simulink model "env_extQ16"  (R2022b)
settings: Solver=VariableStepAuto  StartTime=0.0  StopTime=30  RelTol=1e-3
values from neighbouring files (symbols this model uses):
  B = 8    [variables.m]    (also in variables16.m)
  cordic_delay = 20    [variables.m]    (also in variables16.m)
  e_val = 1/l2    [variables.m]    (also in variables16.m)
  exp_fract_len_homo = 26    [variables.m]    (also in variables16.m = 10)
  exp_word_len_homo = 32    [variables.m]    (also in variables16.m = 16)
  explarge_delay = 3    [variables.m]    (also in variables16.m)
  fft_len_hilb = 2048    [variables.m]    (also in variables16.m)
  fft_length = 4096    [variables.m]    (also in variables16.m)
  frac_bit_l2 = 30    [variables.m]    (also in variables16.m = 14)
  frac_bit_l3 = 29    [variables.m]    (also in variables16.m = 13)
  frac_bit_l4 = 28    [variables.m]    (also in variables16.m = 12)
  grp_delay_hilb = 11    [variables.m]    (also in variables16.m)
  grp_delay_homo = 13    [variables.m]    (also in variables16.m)
  grp_delay_psd = 19    [variables.m]    (also in variables16.m)
  grp_delay_swt = 12    [variables.m]    (also in variables16.m)
  l2 = log(2)    [variables.m]    (also in variables16.m)
  l2e = 1/log2(exp(1))    [variables.m]    (also in variables16.m)
  log2_table = log2((2^(B-1) : 2^(B)) / 2^(B - 1))    [variables.m]    (also in variables16.m)
  log_fract_len_homo = 31    [variables.m]    (also in variables16.m = 15)
  log_latency = 21    [variables.m]    (also in variables16.m)
  log_word_len = 48    [variables.m]    (also in variables16.m = 24)
  log_word_len_homo = 32    [variables.m]    (also in variables16.m = 16)
  NLZLUT = B-ceil(log2((1:2^B)))    [variables.m]    (also in variables16.m)
  scale = 1.0 / (fs * sum(window_val.*window_val))    [variables.m]    (also in variables16.m)
  win_dim = 64    [variables.m]    (also in variables16.m)
  window_dim = 100    [variables.m]    (also in variables16.m)
undefined symbols (not defined in the file or in its folder): C, c, fl_high_index, fl_low_index, HiD, hilbert_fifo_full, LoD, psd_fifo_full, SFVC784, swt_fifo_full, XCK26, xlfda_numerator
libraries: hdlBasic x626, hdlDSPIP x12, hdlUtilities x2, dspsnks4 x1, dspvision x1, vmcUtilities x1
(part 1 of 7)
settings Model: Creator=windows  LastModifiedBy=domen
settings DataIOCC: SaveTime=off

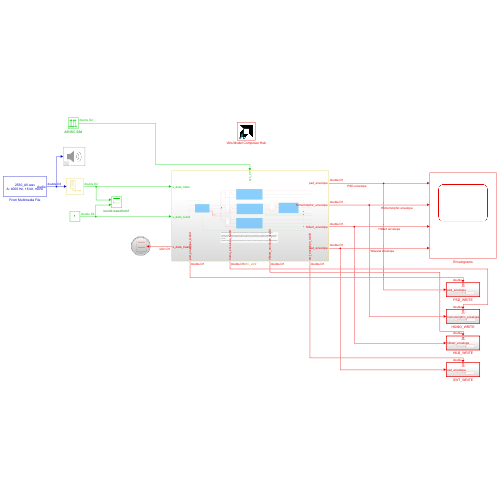
[thumbnail: Simulink's stored preview of the top-level diagram]
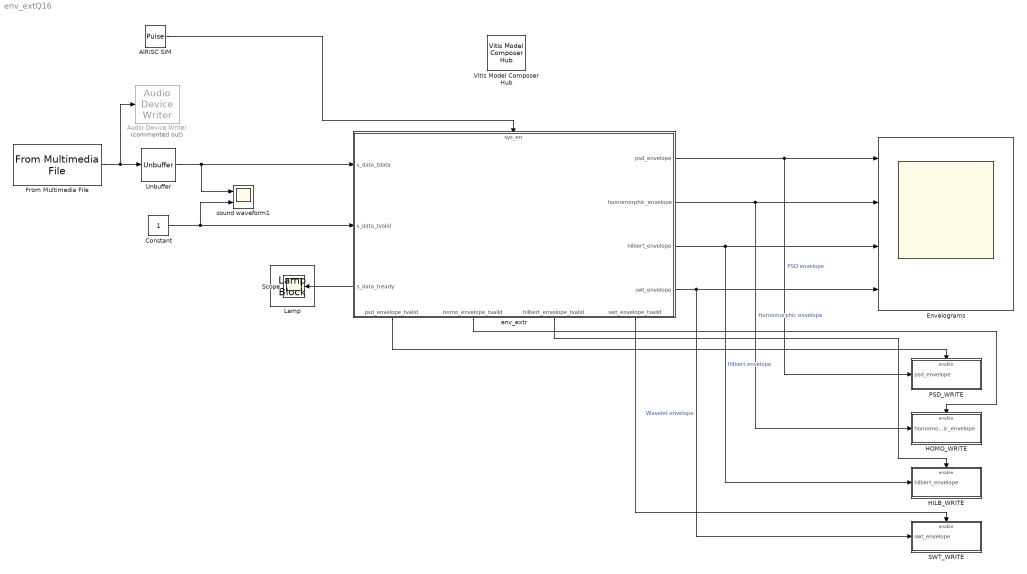
== system env_extQ16 ==
  AIRISC SIM : DiscretePulseGenerator  Period=5120  PulseWidth=2560  PhaseDelay=6144  SampleTime=1/4e3
  Audio Device Writer : dspsnks4/Audio Device Writer  Commented=on  Driver=DirectSound  Device=Default  InheritSampleRate=on  SampleRate=44100  BitDepth=16-bit integer  BufferSize=4096  NumBuffers=10  DefaultOutputChannelMapping=on  OutputChannelMapping=1:2  OutputNumUnderrunSamples=off  DriverIdx=1  DeviceWarnFlag=''
  Constant : Constant  SampleTime=1/4e3
  Envelograms : Scope  NumInputPorts=4
  From Multimedia File : dspvision/From Multimedia File  inputFilename=C:\hss_tests\2530_AV.wav  readRange=[1 Inf]  loop=on  numPlays=1  outputStreams=Audio only  videoDataType=single  audioDataType=double  inheritSampleTime=on  userDefinedSampleTime=1/4  noAudioOutput=off  isIntensityVideo=off  fourcc=RGB  colorVideoFormat=Separate color signals  outputEOF=off  dataOrg=Column-major  audioFrameSize=1024  computeAudioFrameSize=off  outSamplingMode=Sample based
      settings: LibrarySourceBlock=dspsrcs4/From Multimedia File
  HILB_WRITE : Subsystem  TreatAsAtomicUnit=on
  HOMO_WRITE : Subsystem  TreatAsAtomicUnit=on
  Lamp : LampBlock  LabelPosition=Hide
  PSD_WRITE : Subsystem  TreatAsAtomicUnit=on
  SWT_WRITE : Subsystem  TreatAsAtomicUnit=on
  Scope : Scope
  Unbuffer : Unbuffer
  Vitis Model Composer Hub : vmcUtilities/Vitis Model Composer Hub  Tag=genX  CodeGeneration=off  SubsystemName=env_extr  TargetDirectory=./code  ExportType=AI Engines  IpVendor=xilinx.com  IpLibrary=hls  IpVersion=1.0  IpHWLanguage=Verilog  AieCompilerOptions={}  AieSimulatorOptions={}  CreateTestbench=off  TestbenchStackSize=10  RunRtlSim=off  RunCSim=off  RunAieSim=off  AieSimTimeout=50000  RunAieSimProfiling=off  LaunchVitisAnalyzer=off  PlotOutput=off  RunX86Sim=off  X86SimTimeout=10  GenHwImage=off  GenLibadfXo=off  PlatformType=Not Specified  HwSystemType=Baremetal  HwValidationTarget=hw  ProjDevice=Kria KV260 Vision AI Starter Kit (xck26-sfvc784-2LV-c)  ProjDevicePart=XCK26-SFVC784-2LV-C  AIEType=None  SamplePeriod=-1  ClockFrequency=200  DataPathParallelism=1  xilinxfamily=zynquplus  part=xck26  speed=-2LV-c  package=sfvc784  directory=./code\ip\env_extr\src  testbench=off  incr_netlist=off  synthesis_tool=Vivado  clock_wrapper=Clock Enables  dbl_ovrd=According to Block Masks  dcm_input_clock_period=10  sysclk_period=1e9/1e6  simulink_period=1/1e6  eval_field=0  LogFileName=''  NThreads=4
  env_extr : Subsystem
      settings: PortSchema="{\"entries\":[{\"content\":{\"sides\":[{\"content\":{\"connectorIds\":[\"In1\",\"In2\",\"Out9\"]},\"type\":\"ConnectorPlacement.EquallySpacedRectSide\",\"uuid\":\"43992d7e-e6ac-477d-8ccd-89dbeb08d59b\"},{\"content\":{\"connectorIds\":[\"Out1\",\"Out2\",\"Out3\",\"Out4\"],\"side\":\"RIGHT\"},\"type\":\"ConnectorPlacement.EquallySpacedRectSide\",\"uuid\":\"9fd35b87-a22a-4e27-bfaa-04533d92a615\"},{\"content\":{\"connectorIds\":[\"In3\"],\"side\":\"TOP\"},\"type\":\"ConnectorPlacement.EquallySpacedRectSide\",\"uuid\":\"ce144599-82ea-4426-8dad-840a4d497276\"},{\"content\":{\"connectorIds\":[\"Out5\",\"Out6\",\"Out7\",\"Out8\"],\"side\":\"BOTTOM\"},\"type\":\"ConnectorPlacement.EquallySpacedRectSide\",\"uuid\":\"d757f4f1-9e3b-423a-82f0-618de1a239f4\"}]},\"type\":\"ConnectorPlacement.EquallySpacedConnector\",\"uuid\":\"098bbe0e-14d9-4fd5-a746-b1683e211a6b\"}],\"packageUris\":[\"http://schema.mathworks.com/mf0/Connector/R2020b\"],\"version\":\"1.0\"}"
  sound waveform1 : Scope  NumInputPorts=2
  wires:
  env_extr/2(homomorphic_envelope) -> HOMO_WRITE/1(homomorphic_envelope), Envelograms/2  "Homomorphic envelope"
  From Multimedia File/1 -> Unbuffer/1, Audio Device Writer/1
  Unbuffer/1 -> sound waveform1/1, env_extr/1(s_data_tdata)
  env_extr/4(swt_envelope) -> SWT_WRITE/1(swt_envelope), Envelograms/4  "Wavelet envelope"
  env_extr/1(psd_envelope) -> PSD_WRITE/1(psd_envelope), Envelograms/1  "PSD envelope"
  env_extr/3(hilbert_envelope) -> HILB_WRITE/1(hilbert_envelope), Envelograms/3  "Hilbert envelope"
  Constant/1 -> sound waveform1/2, env_extr/2(s_data_tvalid)
  env_extr/9(s_data_tready) -> Scope/1
  env_extr/8(swt_envelope_tvalid) -> SWT_WRITE/Enable
  env_extr/7(hilbert_envelope_tvalid) -> HILB_WRITE/Enable
  env_extr/6(homo_envelope_tvalid) -> HOMO_WRITE/Enable
  env_extr/5(psd_envelope_tvalid) -> PSD_WRITE/Enable
  AIRISC SIM/1 -> env_extr/3(sys_en)

== system env_extQ16/HILB_WRITE ==
  hilbert_envelope : Inport
  Enable : EnablePort
  To Workspace : ToWorkspace  VariableName=hilb_envelope  SampleTime=-1
  wires:
  hilbert_envelope/1 -> To Workspace/1

== system env_extQ16/HOMO_WRITE ==
  homomorphic_envelope : Inport
  Enable : EnablePort
  To Workspace1 : ToWorkspace  VariableName=homo_envelope  SampleTime=-1
  wires:
  homomorphic_envelope/1 -> To Workspace1/1

== system env_extQ16/PSD_WRITE ==
  psd_envelope : Inport
  Enable : EnablePort
  To Workspace3 : ToWorkspace  VariableName=psd_envelope  SampleTime=-1
  wires:
  psd_envelope/1 -> To Workspace3/1

== system env_extQ16/SWT_WRITE ==
  swt_envelope : Inport
  Enable : EnablePort
  To Workspace2 : ToWorkspace  VariableName=swt_envelope  SampleTime=-1
  wires:
  swt_envelope/1 -> To Workspace2/1

== system env_extQ16/env_extr ==
  note: This "feature extractor" system can used to perform the pre-procesing of incoming PCG audio signal.
      |
      | In particular, after a noise removal pre-filtering, it performs, in parallel and in a pipeline fashion, the extraction of four features, namely the PSD envelope, the Hilbert envelope, the Homomorphic envelope and the SWT envelope.
      |
      | The details about the operations performed can be found here: https://ieeexplore.ieee.org/document/7234876
  s_data_tdata : Inport
  s_data_tvalid : Inport  Port=2
  sys_en : Inport  Port=3
  Bus Creator : BusCreator  Inputs=psd_fifo_full,hilbert_fifo_full,swt_fifo_full
  FIFO : hdlBasic/FIFO  mem_type=Block RAM  performance_options=Standard_FIFO  embedded_registers=off  depth=8K  use_asym_data_widths=off  asym_read_width=32  percent_nbits=1  rst=off  rst_latency=2  en=off  use_dcount=off  use_percent_full_port=off  use_almost_empty=off  almost_empty_thresh=3  use_almost_full=off  use_rd_rst_busy=off  use_wr_rst_busy=off  almost_full_thresh=14  almost_empty_offset=[]  almost_full_offset=[]  explicit_period=off  period=[]  store_only_valid=[]  init_zero=[]  simulation_type=fast_sim  XmcBlockStatus=1  maskContainerNames=tabcontainer1  block_type=fifo  block_config=sysgen:FIFO_config  block_width=538  block_height=997
      settings: infoedit=[]
  FIFO1 : hdlBasic/FIFO  mem_type=Block RAM  performance_options=Standard_FIFO  embedded_registers=off  depth=8K  use_asym_data_widths=off  asym_read_width=32  percent_nbits=1  rst=off  rst_latency=2  en=off  use_dcount=off  use_percent_full_port=off  use_almost_empty=off  almost_empty_thresh=2  use_almost_full=off  use_rd_rst_busy=off  use_wr_rst_busy=off  almost_full_thresh=14  almost_empty_offset=[]  almost_full_offset=[]  explicit_period=off  period=[]  store_only_valid=[]  init_zero=[]  simulation_type=fast_sim  XmcBlockStatus=1  maskContainerNames=tabcontainer1  block_type=fifo  block_config=sysgen:FIFO_config  block_width=538  block_height=997
      settings: infoedit=[]
  FIFO2 : hdlBasic/FIFO  mem_type=Block RAM  performance_options=Standard_FIFO  embedded_registers=off  depth=8K  use_asym_data_widths=off  asym_read_width=32  percent_nbits=1  rst=off  rst_latency=2  en=off  use_dcount=off  use_percent_full_port=off  use_almost_empty=off  almost_empty_thresh=3  use_almost_full=off  use_rd_rst_busy=off  use_wr_rst_busy=off  almost_full_thresh=14  almost_empty_offset=[]  almost_full_offset=[]  explicit_period=off  period=[]  store_only_valid=[]  init_zero=[]  simulation_type=fast_sim  XmcBlockStatus=1  maskContainerNames=tabcontainer1  block_type=fifo  block_config=sysgen:FIFO_config  block_width=538  block_height=997
      settings: infoedit=[]
  FIFO3 : hdlBasic/FIFO  mem_type=Block RAM  performance_options=Standard_FIFO  embedded_registers=off  depth=8K  use_asym_data_widths=off  asym_read_width=32  percent_nbits=1  rst=off  rst_latency=2  en=off  use_dcount=off  use_percent_full_port=off  use_almost_empty=off  almost_empty_thresh=1  use_almost_full=off  use_rd_rst_busy=off  use_wr_rst_busy=off  almost_full_thresh=8190  almost_empty_offset=[]  almost_full_offset=[]  explicit_period=off  period=[]  store_only_valid=[]  init_zero=[]  simulation_type=fast_sim  XmcBlockStatus=1  maskContainerNames=tabcontainer1  block_type=fifo  block_config=sysgen:FIFO_config  block_width=538  block_height=997
      settings: infoedit=[]
  FILTERING : Subsystem
      settings: PortSchema="{\"entries\":[{\"content\":{\"sides\":[{\"content\":{\"connectorIds\":[\"In1\",\"In2\",\"Out4\"]},\"type\":\"ConnectorPlacement.EquallySpacedRectSide\",\"uuid\":\"9d039a16-3a48-49d5-80b7-ade04a8e7f96\"},{\"content\":{\"connectorIds\":[\"Out1\",\"Out2\",\"In4\"],\"side\":\"RIGHT\"},\"type\":\"ConnectorPlacement.EquallySpacedRectSide\",\"uuid\":\"bb4be220-296c-4d2d-b90e-a958a467eb47\"},{\"content\":{\"connectorIds\":[\"In3\"],\"side\":\"TOP\"},\"type\":\"ConnectorPlacement.EquallySpacedRectSide\",\"uuid\":\"bb4a24ca-25c4-4b34-8f6b-74df8c85655a\"},{\"content\":{\"connectorIds\":[\"Out3\"],\"side\":\"BOTTOM\"},\"type\":\"ConnectorPlacement.EquallySpacedRectSide\",\"uuid\":\"f96279e1-557f-4274-b1c8-f07939b904f6\"}]},\"type\":\"ConnectorPlacement.EquallySpacedConnector\",\"uuid\":\"a2ca7259-7cd6-4f5b-b082-7ba40fce56a8\"}],\"packageUris\":[\"http://schema.mathworks.com/mf0/Connector/R2020b\"],\"version\":\"1.0\"}"
  HILBERT : Subsystem
      settings: PortSchema="{\"entries\":[{\"content\":{\"sides\":[{\"content\":{\"connectorIds\":[\"In1\",\"In2\",\"Out5\"]},\"type\":\"ConnectorPlacement.EquallySpacedRectSide\",\"uuid\":\"c096cd28-364f-4c7f-b687-c45e0f672067\"},{\"content\":{\"connectorIds\":[\"Out1\",\"Out2\",\"In3\",\"Out3\",\"Out4\",\"In4\"],\"side\":\"RIGHT\"},\"type\":\"ConnectorPlacement.EquallySpacedRectSide\",\"uuid\":\"8f6de1f0-0c6d-47b5-8720-be9e335b7472\"},{\"content\":{\"connectorIds\":[],\"side\":\"TOP\"},\"type\":\"ConnectorPlacement.EquallySpacedRectSide\",\"uuid\":\"cb0bdd80-75cb-433b-a701-3f68d903d9bd\"}]},\"type\":\"ConnectorPlacement.EquallySpacedConnector\",\"uuid\":\"0550c3cb-50ae-4da2-a768-6cf438586d1d\"}],\"packageUris\":[\"http://schema.mathworks.com/mf0/Connector/R2020b\"],\"version\":\"1.0\"}"
  HOMOMORPHIC : Subsystem
      settings: PortSchema="{\"entries\":[{\"content\":{\"sides\":[{\"content\":{\"connectorIds\":[\"In1\",\"In2\",\"Out3\"]},\"type\":\"ConnectorPlacement.EquallySpacedRectSide\",\"uuid\":\"9d039a16-3a48-49d5-80b7-ade04a8e7f96\"},{\"content\":{\"connectorIds\":[\"Out1\",\"Out2\",\"In3\"],\"side\":\"RIGHT\"},\"type\":\"ConnectorPlacement.EquallySpacedRectSide\",\"uuid\":\"bb4be220-296c-4d2d-b90e-a958a467eb47\"},{\"content\":{\"connectorIds\":[],\"side\":\"TOP\"},\"type\":\"ConnectorPlacement.EquallySpacedRectSide\",\"uuid\":\"bb4a24ca-25c4-4b34-8f6b-74df8c85655a\"}]},\"type\":\"ConnectorPlacement.EquallySpacedConnector\",\"uuid\":\"a2ca7259-7cd6-4f5b-b082-7ba40fce56a8\"}],\"packageUris\":[\"http://schema.mathworks.com/mf0/Connector/R2020b\"],\"version\":\"1.0\"}"
      mask Display: %%%%
  PSD : Subsystem
      settings: PortSchema="{\"entries\":[{\"content\":{\"sides\":[{\"content\":{\"connectorIds\":[\"In1\",\"In2\",\"Out3\"]},\"type\":\"ConnectorPlacement.EquallySpacedRectSide\",\"uuid\":\"f634d078-23dc-4ab7-95a0-12deec3a8dc3\"},{\"content\":{\"connectorIds\":[\"Out1\",\"Out2\",\"In3\"],\"side\":\"RIGHT\"},\"type\":\"ConnectorPlacement.EquallySpacedRectSide\",\"uuid\":\"3b518452-2987-4406-a2e9-8ddbf9d6e9f5\"},{\"content\":{\"connectorIds\":[],\"side\":\"TOP\"},\"type\":\"ConnectorPlacement.EquallySpacedRectSide\",\"uuid\":\"9ad2e8b0-6de8-48f9-a4db-ba88e5ff6307\"}]},\"type\":\"ConnectorPlacement.EquallySpacedConnector\",\"uuid\":\"bfdc1522-4211-4337-893d-197f1173dc35\"}],\"packageUris\":[\"http://schema.mathworks.com/mf0/Connector/R2020b\"],\"version\":\"1.0\"}"
  SWT : Subsystem
      settings: PortSchema="{\"entries\":[{\"content\":{\"sides\":[{\"content\":{\"connectorIds\":[\"In1\",\"In2\",\"Out3\"]},\"type\":\"ConnectorPlacement.EquallySpacedRectSide\",\"uuid\":\"9d039a16-3a48-49d5-80b7-ade04a8e7f96\"},{\"content\":{\"connectorIds\":[\"Out1\",\"Out2\",\"In3\"],\"side\":\"RIGHT\"},\"type\":\"ConnectorPlacement.EquallySpacedRectSide\",\"uuid\":\"bb4be220-296c-4d2d-b90e-a958a467eb47\"},{\"content\":{\"connectorIds\":[],\"side\":\"TOP\"},\"type\":\"ConnectorPlacement.EquallySpacedRectSide\",\"uuid\":\"bb4a24ca-25c4-4b34-8f6b-74df8c85655a\"}]},\"type\":\"ConnectorPlacement.EquallySpacedConnector\",\"uuid\":\"a2ca7259-7cd6-4f5b-b082-7ba40fce56a8\"}],\"packageUris\":[\"http://schema.mathworks.com/mf0/Connector/R2020b\"],\"version\":\"1.0\"}"
  psd_envelope : Outport
  homomorphic_envelope : Outport  Port=2
  hilbert_envelope : Outport  Port=3
  swt_envelope : Outport  Port=4
  psd_envelope_tvalid : Outport  Port=5
  homo_envelope_tvalid : Outport  Port=6
  hilbert_envelope_tvalid : Outport  Port=7
  swt_envelope_tvalid : Outport  Port=8
  s_data_tready : Outport  Port=9
  wires:
  SWT/1(m_data_tdata) -> swt_envelope/1
  HOMOMORPHIC/1(m_data_tdata) -> homomorphic_envelope/1
  PSD/1(m_data_tdata) -> psd_envelope/1
  HILBERT/4(hilbert_envelope_data_tdata) -> hilbert_envelope/1
  FILTERING/1(m_data_tdata) -> FIFO1/1, FIFO2/1, FIFO/1
  FILTERING/2(m_data_tvalid) -> FIFO1/2, FIFO/2, FIFO2/2
  FIFO2/1 -> SWT/1(s_data_tdata)
  s_data_tdata/1 -> FILTERING/1(s_data_tdata)
  s_data_tvalid/1 -> FILTERING/2(s_data_tvalid)
  FILTERING/4(s_data_tready) -> s_data_tready/1
  SWT/3(s_data_tready) -> FIFO2/3
  HOMOMORPHIC/3(s_data_tready) -> FIFO3/3
  HILBERT/5(m_data_tready) -> FIFO/3
  HILBERT/1(m_data_tdata) -> FIFO3/1
  HILBERT/2(m_data_tvalid) -> FIFO3/2
  FIFO3/3 -> HILBERT/3(homo_fifo_full_tready)
  PSD/3(s_data_tready) -> FIFO1/3
  FIFO1/1 -> PSD/1(s_data_tdata)
  FIFO1/2 -> PSD/2(s_data_tvalid)
  SWT/2(m_data_tvalid) -> swt_envelope_tvalid/1
  HOMOMORPHIC/2(m_data_tvalid) -> homo_envelope_tvalid/1
  HILBERT/3(hilbert_envelop_data_tvalid) -> hilbert_envelope_tvalid/1
  FIFO/1 -> HILBERT/1(s_data_tdata)
  FIFO/3 -> Bus Creator/2  "hilbert_fifo_full"
  FIFO2/3 -> Bus Creator/3  "swt_fifo_full"
  FIFO2/2 -> SWT/2(s_data_tvalid)
  FIFO/2 -> HILBERT/2(s_data_tvalid)
  FIFO1/3 -> Bus Creator/1  "psd_fifo_full"
  PSD/2(m_data_tvalid) -> psd_envelope_tvalid/1
  Bus Creator/1 -> FILTERING/4(m_data_tready)
  FIFO3/2 -> HOMOMORPHIC/2(s_data_tvalid)
  FIFO3/1 -> HOMOMORPHIC/1(s_data_tdata)
  FILTERING/3(m_ext_tready) -> SWT/3(m_data_ready), HOMOMORPHIC/3(m_data_tready), PSD/3(m_data_ready), HILBERT/4(m_data_ready)
  sys_en/1 -> FILTERING/3(s_ext_tready)

== system env_extQ16/env_extr/FILTERING ==
  note: This stage serves to remove noise from the audio signal.
      | Specifically, a band-pass FIR filter is applied approximating a IIR Butterworth filter which retains frequencies between 25 and 400 Hz.
      | A Schimidt's ( https://github.com/davidspringer/Schmidt-Segmentation-Code/blob/master/schmidt_spike_removal.m ) filter has to be applied to completely remove friction noises but it cannot be used for an online pre-processing setting.
  note: should always be 1, fifo never full.
  s_data_tdata : Inport
  s_data_tvalid : Inport  Port=2
  s_ext_tready : Inport  Port=3
  m_data_tready : Inport  Port=4
  Bus Selector : BusSelector  OutputSignals=psd_fifo_full,hilbert_fifo_full,swt_fifo_full
  FDATool low1 : hdlUtilities/FDATool  block_type=fdatool
      settings: infoedit=FDATool
  FIFO : hdlBasic/FIFO  mem_type=Block RAM  performance_options=Standard_FIFO  embedded_registers=off  depth=256  use_asym_data_widths=off  asym_read_width=32  percent_nbits=1  rst=off  rst_latency=2  en=off  use_dcount=off  use_percent_full_port=off  use_almost_empty=off  almost_empty_thresh=2  use_almost_full=off  use_rd_rst_busy=off  use_wr_rst_busy=off  almost_full_thresh=14  almost_empty_offset=[]  almost_full_offset=[]  explicit_period=off  period=[]  store_only_valid=[]  init_zero=[]  simulation_type=fast_sim  XmcBlockStatus=1  maskContainerNames=tabcontainer1  block_type=fifo  block_config=sysgen:FIFO_config  block_width=538  block_height=997
      settings: infoedit=[]
  FIR Compiler 7.2 : hdlDSPIP/FIR Compiler 7.2   coefficientvector=xlfda_numerator('FDATool low1')  coefficient_sets=1  coefficient_reload=off  filter_type=Single_Rate  rate_change_type=Integer  interpolation_rate=1  decimation_rate=1  zero_pack_factor=1  channel_sequence=Basic  number_channels=1  pattern_list='P4-0,P4-1,P4-2,P4-3,P4-4'  number_paths=1  ratespecification=Input_Sample_Period  sampleperiod=1.00000000  hardwareoversamplingrate=1  coefficient_sign=Signed  quantization=Quantize_Only  coefficient_width=coeff_width  bestprecision=on  coefficient_fractional_bits=33  coefficient_structure=Symmetric  output_rounding_mode=Non_Symmetric_Rounding_Down  output_width=output_width  filter_architecture=Systolic_Multiply_Accumulate  optimization_goal=Area  optimization_list='None'  data_buffer_type=Automatic  coefficient_buffer_type=Automatic  input_buffer_type=Automatic  output_buffer_type=Automatic  preference_for_other_storage=Automatic  multi_column_support=Automatic  columnconfig='41'  inter_column_pipe_length=4  data_has_tlast=Not_Required  m_data_has_tready=on  s_data_has_fifo=on  s_data_has_tuser=Not_Required  m_data_has_tuser=Not_Required  s_config_sync_mode=On_Vector  s_config_method=Single  num_reload_slots=1  has_aclken=off  has_aresetn=off  reset_data_vector=on  trim_axipin_name=off  simulation_type=hybrid_sim  simulation_model=sysgen:xfirv7_2_cmodel  data_path_portlist={ 's_axis_data_tdata', 'm_axis_data_tdata' }  passband_min=0.0  passband_max=0.5  stopband_min=0.5  stopband_max=1.0  filter_selection=1  gui_behaviour='Sysgen_GUI'  data_sign=Signed  data_width=16  data_fractional_bits=0  data_tuser_width=1  wrapper_available=true  ip_wrap_arbitrary_binary_point=true  ip_name=FIR Compiler  ip_version=7.2  dsptool_ready=true  ipcore_usecache=true  ipcore_useipmodelcache=true  port_translation_map={ 'aclken' => 'en', 'aresetn' => 'rst' }  run_core_at_system_period=true  ipcore_xco_need_fpga_part=true  ipcore_fpga_part=[]  XmcBlockStatus=1  maskContainerNames=tabcontainer1  block_type=fir_compiler_v7_2  block_config=sysgen:rodinimport_config  block_width=820  block_height=600
  Inverter : hdlBasic/Inverter  en=off  latency=0  XmcBlockStatus=1  maskContainerNames=group2  block_type=inv  block_config=sysgen:Inverter_config
  Logical : hdlBasic/Logical  logical_function=NAND  inputs=3  en=off  latency=0  precision=Full  arith_type=Unsigned  n_bits=16  bin_pt=0  align_bp=on  overflow=[]  quantization=[]  XmcBlockStatus=1  maskContainerNames=tabcontainer1  block_type=logical  block_config=sysgen:Logical_config
  soc_tready : hdlBasic/Gateway In  gui_display_data_type=Boolean  arith_type=Boolean  n_bits=16  bin_pt=14  preci_type=Single  exp_width=8  frac_width=24  rows=1  columns=1  quantization="Round  (unbiased: +/- Inf)"  overflow=Saturate  period=1/4e3  UseAsADC=off  ADCChannel='1'  interface=None  automatic_assignment=on  address_offset=hex2dec('00')  intf_name=''  intf_description=''  default_value=0  timing_constraint=None  locs_specified=off  LOCs={}  io_standard={}  inherit_from_input=off  hdl_port=on  XmcBlockStatus=1  maskContainerNames=group4  block_type=gatewayin  block_config=sysgen:gateway_in_config  block_width_w=590  block_height_w=620  block_width=640  block_height=850
  steto_in_axis : hdlUtilities/Gateway In AXIS  gui_display_data_type=Fixed-point  arith_type=Signed (2's comp)  n_bits=32  bin_pt=31  preci_type=Custom  exp_width=16  frac_width=24  quantization=Truncate  overflow=Flag as error  OutSampleTime=1/4e3  block_type=gatewayinaxi  XmcBlockStatus=1
  m_data_tdata : Outport
  m_data_tvalid : Outport  Port=2
  m_ext_tready : Outport  Port=3
  s_data_tready : Outport  Port=4
  wires:
  Bus Selector/2 -> Logical/2  "<hilbert_fifo_full>"
  s_data_tdata/1 -> steto_in_axis/1
  s_data_tvalid/1 -> steto_in_axis/2
  steto_in_axis/3 -> s_data_tready/1
  m_data_tready/1 -> Bus Selector/1
  Bus Selector/3 -> Logical/3  "<swt_fifo_full>"
  Bus Selector/1 -> Logical/1  "<psd_fifo_full>"
  Logical/1 -> FIR Compiler 7.2/3
  FIR Compiler 7.2/3 -> m_data_tdata/1
  FIR Compiler 7.2/2 -> m_data_tvalid/1
  s_ext_tready/1 -> soc_tready/1
  soc_tready/1 -> m_ext_tready/1
  steto_in_axis/1 -> FIFO/1
  steto_in_axis/2 -> FIFO/2
  FIR Compiler 7.2/1 -> FIFO/3
  FIFO/1 -> FIR Compiler 7.2/2
  FIFO/2 -> Inverter/1
  Inverter/1 -> FIR Compiler 7.2/1
  FIFO/3 -> steto_in_axis/3
